simulink model "task1"  (R2022b)
settings: Solver=FixedStepAuto  StartTime=0.0  StopTime=7  RelTol=1e-8
undefined symbols (not defined in the file): a0, a1, a2, y0, y1
settings Model: Creator=anton  LastModifiedBy=anton
settings DataIOCC: ExternalInput=data

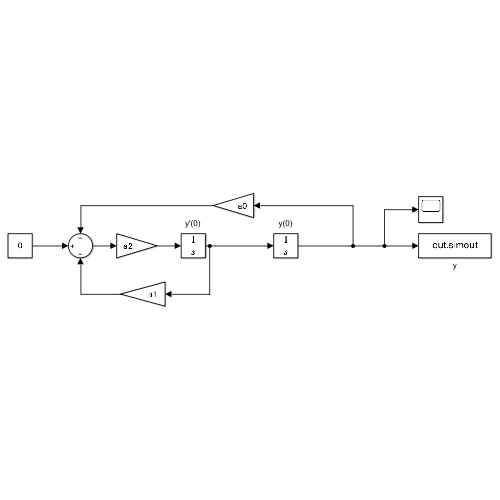
[thumbnail: Simulink's stored preview of the top-level diagram]
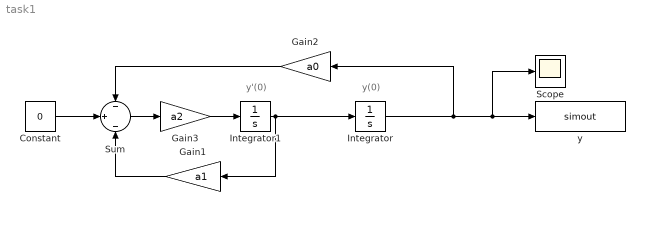
== system task1 ==
  note: y(0)
  note: y'(0)
  Constant : Constant  Value=0
  Gain1 : Gain  Gain=a1
  Gain2 : Gain  Gain=a0
  Gain3 : Gain  Gain=a2
  Integrator : Integrator  InitialCondition=y0
  Integrator1 : Integrator  InitialCondition=y1
  Scope : Scope
  Sum : Sum  Inputs=-|+|-
  y : ToWorkspace  VariableName=simout  SaveFormat=Timeseries  SampleTime=-1
  wires:
  Integrator/1 -> y/1, Scope/1, Gain2/1
  Gain1/1 -> Sum/3
  Integrator1/1 -> Gain1/1, Integrator/1
  Gain3/1 -> Integrator1/1
  Sum/1 -> Gain3/1
  Gain2/1 -> Sum/1
  Constant/1 -> Sum/2
